simulink model "SMPC_safeconstr"  (R2024b)
settings: Solver=ode4  StartTime=0.0  StopTime=tsim  FixedStep=baseRate  RelTol=1e-6  AbsTol=1e-6
values from neighbouring files (symbols this model uses):
  C = [cos(theta), -sin(theta) ... (first row only)    [Run_Initializer.m]
  docking_face = [0 1]'    [Run_Initializer.m]
  docking_offset = [0 0 0]'    [Run_Initializer.m]
  eta = 0.7    [Run_Initializer.m]
  F_t = [kron(eye(N_h),  [zeros(2,3), eye(2), zeros(2,4)]) ... (first row only)    [Run_Initializer.m]
  f_t = [kron(ones(N_h, 1), [xLength yLength]' - edge_buffer) ... (first row only)    [Run_Initializer.m]
  F_u = [kron(eye(N_h),  [eye(3), zeros(3,6)]) ... (first row only)    [Run_Initializer.m]
  f_u = kron(ones(2*N_h, 1), u_max')    [Run_Initializer.m]
  gamma = 0.95    [Run_Initializer.m]
  Gamma1_el = 0.12    [Run_Initializer.m]
  Gamma1_sh = 0.005    [Run_Initializer.m]
  Gamma1_wr = 0.025    [Run_Initializer.m]
  Gamma2_el = 5    [Run_Initializer.m]
  Gamma2_sh = 5    [Run_Initializer.m]
  Gamma2_wr = 5    [Run_Initializer.m]
  Gamma3_el = 10    [Run_Initializer.m]
  Gamma3_sh = 40    [Run_Initializer.m]
  Gamma3_wr = 40    [Run_Initializer.m]
  Gamma4_el = 0.039    [Run_Initializer.m]
  Gamma4_sh = 0.015    [Run_Initializer.m]
  Gamma4_wr = 0.029    [Run_Initializer.m]
  Gamma5_el = 800    [Run_Initializer.m]
  Gamma5_sh = 800    [Run_Initializer.m]
  Gamma5_wr = 800    [Run_Initializer.m]
  Gamma6_el = 0.000001    (= 1e-06)    [Run_Initializer.m]
  Gamma6_sh = 0.005    [Run_Initializer.m]
  Gamma6_wr = 0.02    [Run_Initializer.m]
  H = kron(eye(N_h), [R, zeros(3,6); zeros(6,3), Q])    [Run_Initializer.m]
  Kd_elarm = 0.8    [Run_Initializer.m]
  Kd_sharm = 1.0    (= 1)    [Run_Initializer.m]
  Kd_wrarm = 0.6    [Run_Initializer.m]
  Kp_elarm = 1.2    [Run_Initializer.m]
  Kp_sharm = 1.5    [Run_Initializer.m]
  Kp_wrarm = 1.0    (= 1)    [Run_Initializer.m]
  lambda = (alpha^2)*(6 + kappa) - 6    (= 15.06)    [Run_Initializer.m]
  PWMFreq = 5    [Run_Initializer.m]
  Q_k = [1e-6*eye(3)  zeros(3,3) ... (first row only)    [Run_Initializer.m]
  r_hold_min = [0.8; (0.3+0.05)]    [Run_Initializer.m]
  r_hold_obs = 1.1*sqrt(2)*0.3.*[1;1]    [Run_Initializer.m]
  R_k = diag([0.02^2 0.02^2 0.01^2])    [Run_Initializer.m]
  T_d = 2    [Run_Initializer.m]
  Tz_lim_elarm = .1    (= 0.1)    [Run_Initializer.m]
  Tz_lim_sharm = .1    (= 0.1)    [Run_Initializer.m]
  Tz_lim_wrarm = .1    (= 0.1)    [Run_Initializer.m]
  use_table_constr = false    [Run_Initializer.m]
  w_c = [w_c0, w_i.*ones(1, 2*6)]    [Run_Initializer.m]
  w_m = [w_m0, w_i.*ones(1, 2*6)]    [Run_Initializer.m]
  x_BLACK_0 = [0.32 0.32 315*d2r 0.01 0.005 1*d2r]'    [Run_Initializer.m]
  x_BLUE_0 = [0.5 0.5 315*d2r 0.01 0.01 1*d2r]'    [Run_Initializer.m]
  x_obs_0 = [x_BLUE_0(1:3) + diag(sqrt(R_k)); 0.01; 0.01; 0.005]    [Run_Initializer.m]
  x_tar_0 = [x_BLACK_0(1:3) + diag(sqrt(R_k)); 0.01; 0.01; 0.005]    [Run_Initializer.m]
  zeta = 10*d2r    (= 0.174532925199)    [Run_Initializer.m]
undefined symbols (not defined in the file or in its folder): a1, a2, a3, b0, b1, b2, b3, baseRate, camera_FOV, camera_offset, dataRate, DiscIntNeverNeededParam, drop_states_ARM, drop_states_BLACK, drop_states_BLUE, drop_states_RED, F_black_X_nominal, F_black_Y_nominal, F_blue_X_nominal, F_blue_Y_nominal, F_red_X_nominal, F_red_Y_nominal, F_thrusters_BLACK, F_thrusters_BLUE, F_thrusters_RED, home_states_BLACK, home_states_BLUE, home_states_RED, IBLACK, IBLUE, IDIST, IEE, init_states_BLACK, init_states_BLUE, init_states_RED, IPROX, IRED, K_BLACK, K_BLUE, K_RED, Kd_tb, Kd_tblue, Kd_tr, Kd_xb, Kd_xblue, Kd_xr, Kd_yb, Kd_yblue, Kd_yr, Kp_tb, Kp_tblue, Kp_tr, Kp_xb, Kp_xblue, Kp_xr, Kp_yb, Kp_yblue, Kp_yr, mBLACK, mBLUE ... (+23)
libraries: simulink x30, nvidiaSharedBlocks x12, dspsigops x7, MainLibrary x5, dspinverses x3, nvidiaIMUSensorslib x1
(part 7 of 8)

== matlab function SMPC_safeconstr/PhaseSpace Camera Code/Use Hardware to Obtain States/Store BLACK Data/Subsystem2/Enabled Subsystem/MATLAB Function ==
  data: y input; dy output; dt input; tau input; dy_prev input; ema_prev input; ema output
function [dy, ema] = realtime_derivative_ema(y, dt, tau, dy_prev, ema_prev)
    % Inputs:
    % y: Current measurement
    % dt: Time step
    % alpha: Smoothing factor (e.g., 0.1)

    alpha = 1 - exp(-dt / tau);
        
    % Update EMA
    ema = alpha.*y + (1 - alpha).*ema_prev;
    
    % Compute derivative
    dy = (ema - ema_prev)./dt;
    
end

== matlab function SMPC_safeconstr/PhaseSpace Camera Code/Use Hardware to Obtain States/Store BLUE Data/Calculate True Time Step/MATLAB Function ==
  data: dt input; dt_out output; dataRate input
function dt_out = CheckforInvalidTime(dt, dataRate)

    if dt <= 0

        dt_out = dataRate;

    else

        dt_out = dt;

    end


end

== matlab function SMPC_safeconstr/PhaseSpace Camera Code/Use Hardware to Obtain States/Store BLUE Data/Subsystem1/Enabled Subsystem/MATLAB Function ==
  data: y input; dy output; dt input; tau input; dy_prev input; ema_prev input; ema output
function [dy, ema] = realtime_derivative_ema(y, dt, tau, dy_prev, ema_prev)
    % Inputs:
    % y: Current measurement
    % dt: Time step
    % alpha: Smoothing factor (e.g., 0.1)

    alpha = 1 - exp(-dt / tau);
        
    % Update EMA
    ema = alpha.*y + (1 - alpha).*ema_prev;
    
    % Compute derivative
    dy = (ema - ema_prev)./dt;
    
end

== matlab function SMPC_safeconstr/PhaseSpace Camera Code/Use Hardware to Obtain States/Store BLUE Data/Subsystem2/Enabled Subsystem/MATLAB Function ==
  data: y input; dy output; dt input; tau input; dy_prev input; ema_prev input; ema output
function [dy, ema] = realtime_derivative_ema(y, dt, tau, dy_prev, ema_prev)
    % Inputs:
    % y: Current measurement
    % dt: Time step
    % alpha: Smoothing factor (e.g., 0.1)

    alpha = 1 - exp(-dt / tau);
        
    % Update EMA
    ema = alpha.*y + (1 - alpha).*ema_prev;
    
    % Compute derivative
    dy = (ema - ema_prev)./dt;
    
end

== matlab function SMPC_safeconstr/Simulate Plant Dynamics/RED and ARM Dynamics/RED Only/Dynamics Model for RED/MATLAB Function ==
  data: control_inputs input; x_ddot output; mRED parameter; IRED parameter

    function x_ddot = RED_dynamics(control_inputs, mRED, IRED)

        %#codegen
        % Fully define the size of x_ddot() for code generation:
        x_ddot     = zeros(3,1);

        % Extract the servicer model parameters from the model_param vector defined
        % in initialize.m:

        % Extract the control inputs from the control_input vector:
        Fx        = control_inputs(1);              % [N]
        Fy        = control_inputs(2);              % [N]
        Tz        = control_inputs(3);              % [N.m]

        % Calculate the state acceleration vector:
        x_ddot(1) = Fx/mRED;                      % [m/s^2]
        x_ddot(2) = Fy/mRED;                      % [m/s^2]
        x_ddot(3) = Tz/IRED;                      % [rad/s^2]

    end

== matlab function SMPC_safeconstr/Stochastic Model Predictive Control/Stochastic Model Predictive Control/Execute quadprog ==
  data: z_t input; P input; h input; H parameter; b input; z output; z_0 input; u output; C parameter; result output
% Solve the linear-quadratic optimization problem
function [z, u, result] = fcn(z_t, P, h, H, b, z_0, C)

% Compute equivalent cost function matrices
f = (-2.*z_t'*H)';
H = 2.*H;

% Configure solver options
options = optimoptions('quadprog', 'Algorithm', 'active-set', 'MaxIterations', 300);

% Call solver and time it
tic
[z, ~, exitflag, output] = quadprog(H, f, P, h, C, b, [], [], z_0, options);
cputime = toc;

% Output solver results
result = [exitflag, output.iterations, cputime];

% Extract optimized control input for the current step
u = z(1:3);

== matlab function SMPC_safeconstr/Stochastic Model Predictive Control/Stochastic Model Predictive Control/Propogate BLACK trajectory ==
  data: x_BLACK input; z_BLACK output; T_d parameter
% Compute expected trajectory of the target spacecraft
function z_BLACK = fcn(x_BLACK, T_d)

% Define horizon length
N_h = 15;

% Pre-allocate target trajectory variable
z_BLACK = zeros(9*N_h,1);

% Extract target velocities (assume constant velocity over the horizon)
v_BLACK = x_BLACK(4:6);

% Compute first entry with initial position
z_BLACK(4:9) = [x_BLACK(1:3) + v_BLACK.*T_d; v_BLACK];

% Iterate over the horizon
for j = 2:N_h
    row = 9*(j-1)+1;

    % Extract prior position
    pos_BLACK = z_BLACK(row-9+3:row-9+5);

    % Insert propogated position
    z_BLACK(row+3:row+9-1) = [pos_BLACK + v_BLACK.*T_d; v_BLACK];
end

end

== matlab function SMPC_safeconstr/Stochastic Model Predictive Control/Stochastic Model Predictive Control/Propogate BLUE trajectory ==
  data: x_BLUE input; z_BLUE output; T_d parameter
% Compute expected trajectory of the target spacecraft
function z_BLUE = fcn(x_BLUE, T_d)

% Define horizon length
N_h = 15;

% Pre-allocate target trajectory variable
z_BLUE = zeros(9*N_h,1);

% Extract target velocities (assume constant velocity over the horizon)
v_BLUE = x_BLUE(4:6);

% Compute first entry with initial position
z_BLUE(4:9) = [x_BLUE(1:3) + v_BLUE.*T_d; v_BLUE];

% Iterate over the horizon
for j = 2:N_h
    row = 9*(j-1)+1;

    % Extract prior position
    pos_BLUE = z_BLUE(row-9+3:row-9+5);

    % Insert propogated position
    z_BLUE(row+3:row+9-1) = [pos_BLUE + v_BLUE.*T_d; v_BLUE];
end

end

== matlab function SMPC_safeconstr/Simulate Plant Dynamics/RED and ARM Dynamics/RED + ARM/Data @ Measurement Rate/Calculate True Time Step/MATLAB Function ==
  data: dt input; dt_out output; dataRate input
function dt_out = CheckforInvalidTime(dt, dataRate)

    if dt <= 0

        dt_out = dataRate;

    else

        dt_out = dt;

    end


end

== matlab function SMPC_safeconstr/Simulate Plant Dynamics/RED and ARM Dynamics/RED + ARM/Calculated & Store Measured States/Subsystem3/Enabled Subsystem/MATLAB Function ==
  data: y input; dy output; dt input; tau input; dy_prev input; ema_prev input; ema output
function [dy, ema] = realtime_derivative_ema(y, dt, tau, dy_prev, ema_prev)
    % Inputs:
    % y: Current measurement
    % dt: Time step
    % alpha: Smoothing factor (e.g., 0.1)

    alpha = 1 - exp(-dt / tau);
        
    % Update EMA
    ema = alpha.*y + (1 - alpha).*ema_prev;
    
    % Compute derivative
    dy = (ema - ema_prev)./dt;
    
end

== matlab function SMPC_safeconstr/Stochastic Model Predictive Control/Stochastic Model Predictive Control/Update Holding Radius ==
  data: r_hold input; x_RED input; x_BLACK input; r_hold_min parameter; eta parameter; zeta parameter; gamma parameter; docking_face parameter; r_hold output; docking_offset parameter; docking input; docking output
% Compute next holding radius
function [r_hold, docking] = fcn(r_hold, x_RED, x_BLACK, r_hold_min, eta, zeta, gamma, docking_face, docking_offset, docking)

% Compute 2D z-axis rotation matrix representing the targets attitude
R = [cos(x_BLACK(3)) -sin(x_BLACK(3)); sin(x_BLACK(3)) cos(x_BLACK(3))];

% Compute the docking position in the global frame relative to the target
r_dock = R*(r_hold(2).*docking_face + docking_offset(1:2));

% Compute the required attitude for docking
theta_star = x_BLACK(3) + docking_offset(3)-pi/2;

% Compute required chaser state for docking
x_t = [x_BLACK(1:2) + r_dock; theta_star];

% Compute positional and attitude errors
x_error = (x_RED(1:2) - x_t(1:2))'*(x_RED(1:2) - x_t(1:2));
theta_error = abs(atan2(sin(x_RED(3) - x_t(3)), cos(x_RED(3) - x_t(3))));

% Scale holding radius if tolerances are met
if x_error < eta^2 && theta_error < zeta
    r_hold = gamma*r_hold;
    docking = 1;
end

% Ensure holding radius does go below the defined minimum radius
r_hold = max(r_hold, r_hold_min);

end

== matlab function SMPC_safeconstr/Simulate Plant Dynamics/RED and ARM Dynamics/RED + ARM/Calculated & Store Measured States/Subsystem4/Enabled Subsystem/MATLAB Function ==
  data: y input; dy output; dt input; tau input; dy_prev input; ema_prev input; ema output
function [dy, ema] = realtime_derivative_ema(y, dt, tau, dy_prev, ema_prev)
    % Inputs:
    % y: Current measurement
    % dt: Time step
    % alpha: Smoothing factor (e.g., 0.1)

    alpha = 1 - exp(-dt / tau);
        
    % Update EMA
    ema = alpha.*y + (1 - alpha).*ema_prev;
    
    % Compute derivative
    dy = (ema - ema_prev)./dt;
    
end

== matlab function SMPC_safeconstr/Simulate Plant Dynamics/RED and ARM Dynamics/RED + ARM/Calculated & Store Measured States/Subsystem5/Enabled Subsystem/MATLAB Function ==
  data: y input; dy output; dt input; tau input; dy_prev input; ema_prev input; ema output
function [dy, ema] = realtime_derivative_ema(y, dt, tau, dy_prev, ema_prev)
    % Inputs:
    % y: Current measurement
    % dt: Time step
    % alpha: Smoothing factor (e.g., 0.1)

    alpha = 1 - exp(-dt / tau);
        
    % Update EMA
    ema = alpha.*y + (1 - alpha).*ema_prev;
    
    % Compute derivative
    dy = (ema - ema_prev)./dt;
    
end

== matlab function SMPC_safeconstr/Stochastic Model Predictive Control/Unscented Kalman Filter (TARGET)/Unscented Kalman Filter ==
  data: x_0 input; P_0 input; z input; x_est output; P_est output; baseRate parameter; Q_k parameter; R_k parameter; lambda parameter; w_m parameter; w_c parameter
function [x_est, P_est] = fcn(x_0, P_0, z, baseRate, Q_k, R_k, lambda, w_m, w_c)
    % Define dynamics model (using forward euler integration)
    dynamics = @(x, dt) x + dt.*[x(4:6); zeros(3,1)];

    % Define measurement model
    measure = @(x) x(1:3);

    % Run a step of the UKF
    [x_est, P_est] = estimate_UKF(x_0, P_0, z, baseRate, dynamics, measure, ...
                                  6, Q_k, R_k, lambda, w_m, w_c, 3);
end

%% Unscented Kalman Filter Estimation
function [x_est, P_est] = estimate_UKF(x_0, P_0, z, dt, dynamics_fcn, measure_fcn, N, Q, R, lambda, w_m, w_c, d_max)
    % Compute the cholesky decomposition
    L = chol((N + lambda)*P_0)';
    
    % Place sigma points
    X = [x_0, x_0 + L, x_0 - L];
    
    % Propogate sigma points through the dynamics model
    X_plus = zeros(size(X));
    for i = 1:size(X,2)
        X_plus(:,i) = dynamics_fcn(X(:,i), dt);
    end

    % Compute the predicted state and covariance
    x_bar = X_plus*w_m';
    P_bar = (X_plus - x_bar)*diag(w_c)*(X_plus - x_bar)' + Q;

    % Transfer sigma points into the measurement space
    Z = zeros(size(z,1), size(X,2));
    for i = 1:size(X,2)
        Z(:,i) = measure_fcn(X_plus(:,i));
    end

    % Compute the predicted measurement
    z_bar = Z*w_m';

    % Compute measurement covariance and state-measurement cross-covariance
    P_zz = (Z - z_bar)*diag(w_c)*(Z - z_bar)' + R;
    P_xz = (X_plus - x_bar)*diag(w_c)*(Z - z_bar)';

    % Compute the residue
    y = z - z_bar;

    if anynan(z) || all(z == 0) || y'*P_zz*y >= d_max^2
        % If there is no measurement, or it is an outlier, use prediction only
        x_est = x_bar;
        P_est = P_bar;
    else
        % Compute the kalman gain
        % K = P_xz/P_zz;
        K = P_xz*inv(P_zz);

        % Compute estimated state and covariance
        x_est = x_bar + K*y;
        P_est = P_bar - K*P_zz*K';
    end
end

== matlab function SMPC_safeconstr/Stochastic Model Predictive Control/Stochastic Model Predictive Control/Obstacle Collision Constraint ==
  data: r_hold_obs parameter; z_BLUE input; F_c output; z_RED input; f_c output; platformSelection parameter; P input
function [F_c, f_c] = fcn(r_hold_obs, z_BLUE, z_RED, platformSelection, P)

% Define horizon length
N_h = 15;

% Define shape matrix
S = diag(r_hold_obs.^-2);

% Pre-allocate expansion point position vector over the horizon
r_0_bar = zeros(9*N_h,1);

% Pre-allocate D matrix
F_c = zeros(N_h, 9*N_h);
f_c = zeros(N_h,1);

alpha = zeros(N_h,1);

if platformSelection >= 6 && platformSelection <= 11
    
    % Iterate over the horizon
    for j = 1:N_h
        pos = 9*(j-1)+1;
        
        % Extract target & chaser positions, and target attitude
        r_obs = z_BLUE(pos+3:pos+4);
        r_chs = z_RED(pos+3:pos+4);
        theta_tar = z_BLUE(pos+5);
    
        % Compute target -> chaser unit vector
        u_tc = (r_chs-r_obs)/norm(r_chs-r_obs);
    
        % Compute target body-fixed -> inertial rotation matrix
        R = [cos(theta_tar) -sin(theta_tar); 
             sin(theta_tar) cos(theta_tar)];
    
        % Compute angle between target-chaser vector and target body-fixed
        % x-axis in inertial frame
        theta_e = acos(u_tc'*(R*[1; 0]));
    
        % Extract semi-(major/minor) axes
        [a_e, b_e] = deal(r_hold_obs(1), r_hold_obs(2));
    
        % Compute ellipse radius at current angle
        r_e = a_e*b_e/sqrt((a_e*sin(theta_e))^2 + (b_e*cos(theta_e))^2);
    
        % Compute expansion point position
        r_0 = r_obs + r_e.*u_tc;
    
        % Store expansion point positions in respective vector
        r_0_bar(pos+3:pos+4) = r_0;
    
        % Configure solver options
        options = optimoptions('quadprog', 'Algorithm', 'active-set', 'MaxIterations', 300);

        w = diag(P(1:2,1:2));

        % Call solver and time it
        w_opt = quadprog(2.*(R*S*R'), (2.*(r_obs-r_chs)'*(R*S*R'))', [], [], [], [], -w, w, [0 0], options);
        alpha(j) = w_opt'*(R*S*R')*w_opt+2*(r_obs-r_chs)'*(R*S*R')*w_opt;

        % Compute E matrix
        E = (r_0-r_obs)'*(R*S*R');
    
        row = j;
        col = 3+9*(j-1)+1;
        
        F_c(row,col:col+1) = -2.*E;
        f_c(row,1) = -1-E*(r_0+r_obs); %+ alpha(j);
    
    end
end

end

== matlab function SMPC_safeconstr/2 - Guidance/Default APF PPL (BLACK)/MATLAB Function ==
  data: desiredPosition input; currentPosition output; currentPosition input; obstacles input; attractiveGain input; repulsiveGain input; influenceRange input; angularGain input; baseRate parameter
function currentPosition = APFPathPlanner(desiredPosition, currentPosition, obstacles, attractiveGain, repulsiveGain, influenceRange, angularGain, baseRate)
    % APFPathPlanner for real-time path planning in Simulink
    % Controls X, Y, and Attitude (Theta)
    % currentPosition: [x, y, theta]
    % desiredPosition: [x, y, theta]
    % obstacles: Nx2 matrix of obstacle positions [x, y]
    % attractiveGain: Scalar for attractive force
    % repulsiveGain: Scalar for repulsive force
    % influenceRange: Scalar, range for obstacle influence
    % angularGain: Scalar for angular adjustment


    % Position control for X and Y
    attractiveForce = attractiveGain * (desiredPosition(1:2) - currentPosition(1:2));
    repulsiveForce = zeros(1, 2);

    % % Repulsive force from obstacles
    for i = 1:size(obstacles, 1)
        obstaclePos = obstacles(i, :);
        distanceToObstacle = norm(currentPosition(1:2) - obstaclePos);

        if distanceToObstacle < influenceRange
            directionFromObstacle = (currentPosition(1:2) - obstaclePos) / distanceToObstacle;
            magnitude = repulsiveGain * (1 / distanceToObstacle - 1 / influenceRange) * (1 / distanceToObstacle^2);
            repulsiveForce = repulsiveForce + magnitude * directionFromObstacle;
        end
    end

    % Combine attractive and repulsive forces
    totalForce = attractiveForce + repulsiveForce;

    % Update X and Y position
    deltaT = baseRate;
    newPosition = currentPosition(1:2) + deltaT * totalForce;

    % Attitude control for Theta
    angularDifference = atan2(sin(desiredPosition(3) - currentPosition(3)), cos(desiredPosition(3) - currentPosition(3)));
    newTheta = currentPosition(3) + angularGain * angularDifference * deltaT;

    % Normalize newTheta to be within -pi to pi
    newTheta = atan2(sin(newTheta), cos(newTheta));

    % Update currentPosition with new position and attitude
    currentPosition = [newPosition, newTheta];

end

== matlab function SMPC_safeconstr/Stochastic Model Predictive Control/Stochastic Model Predictive Control/Target Vision Constraint ==
  data: z_BLACK input; z_RED input; docking input; f_v output; docking_offset parameter; camera_FOV parameter; camera_offset parameter
 function f_v = fcn(z_BLACK, z_RED, docking, docking_offset, camera_FOV, camera_offset)

% Define horizon length
N_h = 15;

% Pre-allocate p vector
f_v = zeros(2*N_h,1);

% Iterate over the horizon
for j = 1:N_h
    pos = 9*(j-1)+1;

    R = [cos(z_RED(pos+5)), -sin(z_RED(pos+5)); 
         sin(z_RED(pos+5)),  cos(z_RED(pos+5))];

    % Compute relative position vector from camera to target
    r = z_BLACK(pos+3:pos+4) - z_RED(pos+3:pos+4) + R*camera_offset;

    % Compute desired pointing angle
    theta_star = rotateToFace(z_RED(pos+5), r) + docking_offset(3);

    if docking
        f_v(j) = theta_star + pi;
        f_v(j+N_h) = -1*(theta_star - pi);
    else
        f_v(j) = theta_star + (camera_FOV/2);
        f_v(j+N_h) = -1*(theta_star - (camera_FOV/2));
    end
end

end

%% Functions

function theta_des = rotateToFace(theta, r)
    theta_des = theta + wrapToPi(atan2(r(2),r(1)) - theta);
end

== matlab function SMPC_safeconstr/Thruster Control Code/Change BLACK Behavior/Calculate Duty Cycle/Generate Initial Guess/MATLAB Function ==
  data: H output; thruster_dist2CG_BLACK parameter; F_thrusters_BLACK parameter
function H = MakeH(thruster_dist2CG_BLACK,F_thrusters_BLACK)

    Vec1 = [ -1
             -1
              0 
              0
              1
              1
              0
              0 ];
          
    Vec2 = [  0
              0
              1
              1
              0
              0
             -1
             -1 ];
         
    Vec3 = thruster_dist2CG_BLACK./1000;
    
    Mat1 = [Vec1, Vec2, Vec3]';
    
    Mat2 = diag((F_thrusters_BLACK./2));
    
    H    = Mat1*Mat2;

end

== matlab function SMPC_safeconstr/Corrupt Ground Truth/Custom Noise Generator ==
  data: y output; u parameter; v parameter
function y = fcn(u, v)
    if length(u) ~= length(v)
        error('The length of the means and variances must be the same')
    end
    
    y = u + sqrt(v).*randn(length(u),1);
end

== matlab function SMPC_safeconstr/Thruster Control Code/Change BLACK Behavior/Calculate Duty Cycle/MATLAB Function1 ==
  data: ThrustPer_Final output; ThrustPer input; PWMFreq parameter
function ThrustPer_Final  = ThrusterSat(ThrustPer, PWMFreq)

    ValveTime       = 0.007;
    TControl        = 1/PWMFreq;

    ThrustPer_Final = zeros(8,1);
    
    if max(ThrustPer) > 1
        ThrustPer_Sat = ThrustPer/max(ThrustPer);
    else
        ThrustPer_Sat = ThrustPer;
    end
    
    for i = 1:8
        if ThrustPer_Sat(i) > ValveTime/TControl 
            ThrustPer_Final(i) = ThrustPer_Sat(i);
        else
            %ThrustPer_Final(i) = 0;
        end
    end


end

== matlab function SMPC_safeconstr/Corrupt Ground Truth/Custom Noise Generator1 ==
  data: y output; u parameter; v parameter
function y = fcn(u, v)
    if length(u) ~= length(v)
        error('The length of the means and variances must be the same')
    end
    
    y = u + sqrt(v).*randn(length(u),1);
end

== matlab function SMPC_safeconstr/Stochastic Model Predictive Control/Stochastic Model Predictive Control/Compute Target Trajectory ==
  data: r_hold input; z_RED input; z_BLACK input; docking input; docking_face parameter; z_t output; docking_offset parameter
% Compute docking position over the horizon
function z_t  = fcn(r_hold, z_RED, z_BLACK, docking, docking_face, docking_offset)

% Define horizon length
N_h = 15;

% Pre-allocate target trajectory vector
z_t = zeros(9*N_h,1);

% Iterate over the horizon
for j = 1:N_h
    pos = 9*(j-1)+1;
    % Compute 2D z-axis rotation matrix representing the targets attitude
    R = rotz(z_BLACK(pos+5));

    % Compute the docking position in the global frame relative to the target
    r_dock = R*(r_hold(2).*docking_face + docking_offset(1:2));

    % Compute the required attitude for docking
        
    theta_star = z_BLACK(pos+5) + docking_offset(3)-pi/2;
    
    % Store required attitude and position for docking
    z_t(pos+3:pos+4) = z_BLACK(pos+3:pos+4) + r_dock;
    z_t(pos+5) = theta_star;
end

end

%% Functions

function C = rotz(theta)
    C = [cos(theta) -sin(theta); sin(theta) cos(theta)];
end

function theta_des = rotateToFace(theta, r)
    theta_des = theta + wrapToPi(atan2(r(2),r(1)) - theta);
end

== matlab function SMPC_safeconstr/Stochastic Model Predictive Control/Stochastic Model Predictive Control/Dynamic Target Collision Constraint ==
  data: r_hold input; z_BLACK input; F_h output; z_RED input; f_h output; P input
function [F_h, f_h] = fcn(r_hold, z_BLACK, z_RED, P)

% Define horizon length
N_h = 15;

% Define shape matrix
S = diag(r_hold.^-2);

% Pre-allocate expansion point position vector over the horizon
r_0_bar = zeros(9*N_h,1);

% Pre-allocate D matrix
F_h = zeros(N_h, 9*N_h);
f_h = zeros(N_h,1);

alpha = zeros(N_h,1);

% Iterate over the horizon
for j = 1:N_h
    pos = 9*(j-1)+1;
    
    % Extract target & chaser positions, and target attitude
    r_tar = z_BLACK(pos+3:pos+4);
    r_chs = z_RED(pos+3:pos+4);
    theta_tar = z_BLACK(pos+5);

    % Compute target -> chaser unit vector
    u_tc = (r_chs-r_tar)/norm(r_chs-r_tar);

    % Compute target body-fixed -> inertial rotation matrix
    R = [cos(theta_tar) -sin(theta_tar); 
         sin(theta_tar) cos(theta_tar)];

    % Compute angle between target-chaser vector and target body-fixed
    % x-axis in inertial frame
    theta_e = acos(u_tc'*(R*[1; 0]));

    % Extract semi-(major/minor) axes
    [a_e, b_e] = deal(r_hold(1), r_hold(2));

    % Compute ellipse radius at current angle
    r_e = a_e*b_e/sqrt((a_e*sin(theta_e))^2 + (b_e*cos(theta_e))^2);

    % Compute expansion point position
    r_0 = r_tar + r_e.*u_tc;

    % Store expansion point positions in respective vector
    r_0_bar(pos+3:pos+4) = r_0;

    % Configure solver options
    options = optimoptions('quadprog', 'Algorithm', 'active-set', 'MaxIterations', 300);
    
    w = diag(P(1:2,1:2));

    % Call solver and time it
    w_opt = quadprog(2.*(R*S*R'), (2.*(r_tar-r_chs)'*(R*S*R'))', [], [], [], [], -w, w, [0 0], options);
    alpha(j) = w_opt'*(R*S*R')*w_opt+2*(r_tar-r_chs)'*(R*S*R')*w_opt;

    % Compute E matrix
    E = (r_0-r_tar)'*(R*S*R');

    row = j;
    col = 3+9*(j-1)+1;

    F_h(row,col:col+1) = -2.*E;
    f_h(row) = -1-E*(r_0+r_tar);% + alpha(j);

end

r_tar = z_BLACK(4:5);
r_chs = z_RED(4:5);
u_tc = (r_chs-r_tar)/norm(r_chs-r_tar);

out = [f_h(1) r_tar' u_tc' z_BLACK(6) alpha(1)];

end

== matlab function SMPC_safeconstr/Stochastic Model Predictive Control/Stochastic Model Predictive Control/Shift Optimization Variable ==
  data: z input; z_0 output
function z_0 = fcn(z)

% Shift reference trajectory by dropping first control input and state,
% set last control input as zeros and duplicate last state
z_0 = [z(9+1:end); zeros(3,1); z(end-5:end)];

end

== matlab function SMPC_safeconstr/Thruster Control Code/Change BLACK Behavior/Calculate Duty Cycle/MATLAB Function5 ==
  data: H_final output; u_desired input; duty_cycles output; x0 input; thruster_dist2CG_BLACK parameter; F_black_X_nominal parameter; F_black_Y_nominal parameter; max_iters parameter; tol parameter
function [H_final,duty_cycles] = optimize_duty_cycle_with_decay(u_desired, x0, thruster_dist2CG_BLACK, F_black_X_nominal, F_black_Y_nominal, max_iters, tol)
    % Optimizes thruster duty cycles with decay factor updates
    %
    % Inputs:
    %   u_desired - Desired force and torque vector [Fx; Fy; M] (3x1)
    %   x0 - Initial guess for duty cycles (vector, 8x1)
    %   max_iters - Maximum number of iterations for convergence
    %   tol - Convergence tolerance for duty cycles
    %   thruster_dist2CG_BLACK - Distances of thrusters from CG (vector, mm)
    %   F_red_X_nominal - Nominal X thruster force (scalar, N)
    %   F_red_Y_nominal - Nominal Y thruster force (scalar, N)
    %
    % Outputs:
    %   duty_cycles - Optimal duty cycles for each thruster (vector, 8x1)

    % Initialization
    num_thrusters = length(x0);
    duty_cycles = x0; % Start with the initial guess
    thrust_decay_factor = 1; % Initial decay factor
    prev_duty_cycles = duty_cycles + 2 * tol; % Ensure loop starts

    % Iterative optimization process
    for iter = 1:max_iters
        % Update H matrix based on the current decay factor
        H = MakeHWithDecay(thruster_dist2CG_BLACK, F_black_X_nominal, thrust_decay_factor, F_black_Y_nominal);
        
        % Define quadratic programming problem
        Q = 2 * (H' * H); % Quadratic term
        c = -2 * (H' * u_desired); % Linear term
        lb = zeros(num_thrusters, 1); % Lower bounds
        ub = ones(num_thrusters, 1); % Upper bounds
        options = optimoptions('quadprog', 'Display', 'off', 'Algorithm', 'active-set', 'MaxIterations', 5);
        
        % Solve for optimal duty cycles
        [duty_cycles, ~, ~] = quadprog(Q, c, [], [], [], [], lb, ub, duty_cycles, options);
        
        % Update decay factor based on the current duty cycles
        [thrust_decay_factor, ~] = check_thrust_decay(duty_cycles);
                
        % Check convergence criteria
        if norm(duty_cycles - prev_duty_cycles, Inf) < tol
            H_final = MakeHWithDecayRecalculateForce(thruster_dist2CG_BLACK, F_black_X_nominal, thrust_decay_factor, F_black_Y_nominal);
            return;
        end
            
        
        % Update for next iteration
        prev_duty_cycles = duty_cycles;
    end
    
    H_final = MakeHWithDecayRecalculateForce(thruster_dist2CG_BLACK, F_black_X_nominal, thrust_decay_factor, F_black_Y_nominal);
   

end

function H = MakeHWithDecay(thruster_dist2CG, F_X_nominal, thrust_decay_factor, F_Y_nominal)
    % Constructs the H matrix with thrust decay adjustments
    %
    % Inputs:
    %   thruster_dist2CG - Distances of thrusters from CG (vector, mm)
    %   F_X_nominal - Nominal X thruster force (scalar, N)
    %   thrust_decay_factor - Decay factor for thrust (scalar)
    %   F_Y_nominal - Nominal Y thruster force (scalar, N)
    %
    % Output:
    %   H - H matrix for optimization (3x8)

    % Adjust thruster distances (convert to meters)
    adjusted_thruster_dist2CG = thruster_dist2CG / 1000;

    % Define thruster contribution vectors
    Vec1 = [-1; -1;  0;  0;  1;  1;  0;  0]; % X-component
    Vec2 = [ 0;  0;  1;  1;  0;  0; -1; -1]; % Y-component
    Vec3 = adjusted_thruster_dist2CG;        % Moment arm (Z)

    % Combine vectors into the H matrix structure
    Mat1 = [Vec1, Vec2, Vec3]';
    
    % Adjust thruster forces with decay factor
    F_thrusters = [F_X_nominal; F_X_nominal; F_Y_nominal; F_Y_nominal; 
                   F_X_nominal; F_X_nominal; F_Y_nominal; F_Y_nominal] * thrust_decay_factor;

    % Scale forces for H matrix
    Mat2 = diag(F_thrusters / 2);

    % Compute final H matrix
    H = Mat1 * Mat2;
end

function H = MakeHWithDecayRecalculateForce(thruster_dist2CG, F_X_nominal, thrust_decay_factor, F_Y_nominal)
    % Constructs the H matrix with thrust decay adjustments
    %
    % Inputs:
    %   thruster_dist2CG - Distances of thrusters from CG (vector, mm)
    %   F_X_nominal - Nominal X thruster force (scalar, N)
    %   thrust_decay_factor - Decay factor for thrust (scalar)
    %   F_Y_nominal - Nominal Y thruster force (scalar, N)
    %
    % Output:
    %   H - H matrix for optimization (3x8)

    % Adjust thruster distances (convert to meters)
    adjusted_thruster_dist2CG = thruster_dist2CG / 1000;

    % Define thruster contribution vectors
    Vec1 = [-1; -1;  0;  0;  1;  1;  0;  0]; % X-component
    Vec2 = [ 0;  0;  1;  1;  0;  0; -1; -1]; % Y-component
    Vec3 = adjusted_thruster_dist2CG;        % Moment arm (Z)

    % Combine vectors into the H matrix structure
    Mat1 = [Vec1, Vec2, Vec3]';
    
    % Adjust thruster forces with decay factor
    F_thrusters = [F_X_nominal; F_X_nominal; F_Y_nominal; F_Y_nominal; 
                   F_X_nominal; F_X_nominal; F_Y_nominal; F_Y_nominal] * thrust_decay_factor;

    % Scale forces for H matrix
    Mat2 = diag(F_thrusters);

    % Compute final H matrix
    H = Mat1 * Mat2;
end

function [thrust_decay_factor, count] = check_thrust_decay(PWMs)
    % Updates the thrust decay factor based on current duty cycles
    %
    % Inputs:
    %   PWMs - Current duty cycle values (vector)
    %
    % Outputs:
    %   thrust_decay_factor - Updated decay factor (scalar)
    %   count - Number of active thrusters (scalar)

    % Normalize PWMs if necessary
    if max(PWMs) > 1
        PWMs = PWMs / max(PWMs);
    end

    % Count active thrusters
    count = sum(PWMs > 0);
    
    % Compute average duty cycle for active thrusters
    average_duty_cycle_per_thruster = sum(max(PWMs, 0)) / max(count, 1);

    % Update thrust decay factor based on average duty cycle
    if average_duty_cycle_per_thruster < 0.3 || count == 0
        thrust_decay_factor = 1;
    else
        thrust_decay_factor = max(0.6 - 2 * average_duty_cycle_per_thruster + 1, 0.5);
    end
end

== matlab function SMPC_safeconstr/Thruster Control Code/Change BLACK Behavior/Calculate Duty Cycle/Rotate Forces to Inertial/Create Rotation Matrix ==
  data: Rz input; C_Ib output
function C_Ib = RotateFrame(Rz)

C_bI = [  cos(Rz) sin(Rz)
         -sin(Rz) cos(Rz) ];

C_Ib = inv(C_bI);

end

== matlab function SMPC_safeconstr/Thruster Control Code/Change BLACK Behavior/Rotate Forces to Body/Create Rotation Matrix ==
  data: Rz input; C_bI output
function C_bI = RotateFrame(Rz)

C_bI = [  cos(Rz) sin(Rz)
         -sin(Rz) cos(Rz) ];

end

== matlab function SMPC_safeconstr/Thruster Control Code/Change BLUE Behavior/Calculate Duty Cycle/Generate Initial Guess/MATLAB Function ==
  data: H output; thruster_dist2CG_BLUE parameter; F_thrusters_BLUE parameter
function H = MakeH(thruster_dist2CG_BLUE,F_thrusters_BLUE)

    Vec1 = [ -1
             -1
              0 
              0
              1
              1
              0
              0 ];
          
    Vec2 = [  0
              0
              1
              1
              0
              0
             -1
             -1 ];
         
    Vec3 = thruster_dist2CG_BLUE./1000;
    
    Mat1 = [Vec1, Vec2, Vec3]';
    
    Mat2 = diag((F_thrusters_BLUE./2));
    
    H    = Mat1*Mat2;

end

== matlab function SMPC_safeconstr/Thruster Control Code/Change BLUE Behavior/Calculate Duty Cycle/MATLAB Function1 ==
  data: ThrustPer_Final output; ThrustPer input; PWMFreq parameter
function ThrustPer_Final  = ThrusterSat(ThrustPer, PWMFreq)

    ValveTime       = 0.007;
    TControl        = 1/PWMFreq;

    ThrustPer_Final = zeros(8,1);
    
    if max(ThrustPer) > 1
        ThrustPer_Sat = ThrustPer/max(ThrustPer);
    else
        ThrustPer_Sat = ThrustPer;
    end
    
    for i = 1:8
        if ThrustPer_Sat(i) > ValveTime/TControl 
            ThrustPer_Final(i) = ThrustPer_Sat(i);
        else
            ThrustPer_Final(i) = 0;
        end
    end


end

== matlab function SMPC_safeconstr/Thruster Control Code/Change BLUE Behavior/Calculate Duty Cycle/MATLAB Function5 ==
  data: H_final output; u_desired input; duty_cycles output; x0 input; thruster_dist2CG_BLUE parameter; F_blue_X_nominal parameter; F_blue_Y_nominal parameter; max_iters parameter; tol parameter
function [H_final,duty_cycles] = optimize_duty_cycle_with_decay(u_desired, x0, thruster_dist2CG_BLUE, F_blue_X_nominal, F_blue_Y_nominal, max_iters, tol)
    % Optimizes thruster duty cycles with decay factor updates
    %
    % Inputs:
    %   u_desired - Desired force and torque vector [Fx; Fy; M] (3x1)
    %   x0 - Initial guess for duty cycles (vector, 8x1)
    %   max_iters - Maximum number of iterations for convergence
    %   tol - Convergence tolerance for duty cycles
    %   thruster_dist2CG_BLUE - Distances of thrusters from CG (vector, mm)
    %   F_red_X_nominal - Nominal X thruster force (scalar, N)
    %   F_red_Y_nominal - Nominal Y thruster force (scalar, N)
    %
    % Outputs:
    %   duty_cycles - Optimal duty cycles for each thruster (vector, 8x1)

    % Initialization
    num_thrusters = length(x0);
    duty_cycles = x0; % Start with the initial guess
    thrust_decay_factor = 1; % Initial decay factor
    prev_duty_cycles = duty_cycles + 2 * tol; % Ensure loop starts

    % Iterative optimization process
    for iter = 1:max_iters
        % Update H matrix based on the current decay factor
        H = MakeHWithDecay(thruster_dist2CG_BLUE, F_blue_X_nominal, thrust_decay_factor, F_blue_Y_nominal);
        
        % Define quadratic programming problem
        Q = 2 * (H' * H); % Quadratic term
        c = -2 * (H' * u_desired); % Linear term
        lb = zeros(num_thrusters, 1); % Lower bounds
        ub = ones(num_thrusters, 1); % Upper bounds
        options = optimoptions('quadprog', 'Display', 'off', 'Algorithm', 'active-set', 'MaxIterations', 5);
        
        % Solve for optimal duty cycles
        [duty_cycles, ~, ~] = quadprog(Q, c, [], [], [], [], lb, ub, duty_cycles, options);
        
        % Update decay factor based on the current duty cycles
        [thrust_decay_factor, ~] = check_thrust_decay(duty_cycles);
                
        % Check convergence criteria
        if norm(duty_cycles - prev_duty_cycles, Inf) < tol
            H_final = MakeHWithDecayRecalculateForce(thruster_dist2CG_BLUE, F_blue_X_nominal, thrust_decay_factor, F_blue_Y_nominal);
            return;
        end
            
        
        % Update for next iteration
        prev_duty_cycles = duty_cycles;
    end
    
    H_final = MakeHWithDecayRecalculateForce(thruster_dist2CG_BLUE, F_blue_X_nominal, thrust_decay_factor, F_blue_Y_nominal);
   

end

function H = MakeHWithDecay(thruster_dist2CG, F_X_nominal, thrust_decay_factor, F_Y_nominal)
    % Constructs the H matrix with thrust decay adjustments
    %
    % Inputs:
    %   thruster_dist2CG - Distances of thrusters from CG (vector, mm)
    %   F_X_nominal - Nominal X thruster force (scalar, N)
    %   thrust_decay_factor - Decay factor for thrust (scalar)
    %   F_Y_nominal - Nominal Y thruster force (scalar, N)
    %
    % Output:
    %   H - H matrix for optimization (3x8)

    % Adjust thruster distances (convert to meters)
    adjusted_thruster_dist2CG = thruster_dist2CG / 1000;

    % Define thruster contribution vectors
    Vec1 = [-1; -1;  0;  0;  1;  1;  0;  0]; % X-component
    Vec2 = [ 0;  0;  1;  1;  0;  0; -1; -1]; % Y-component
    Vec3 = adjusted_thruster_dist2CG;        % Moment arm (Z)

    % Combine vectors into the H matrix structure
    Mat1 = [Vec1, Vec2, Vec3]';
    
    % Adjust thruster forces with decay factor
    F_thrusters = [F_X_nominal; F_X_nominal; F_Y_nominal; F_Y_nominal; 
                   F_X_nominal; F_X_nominal; F_Y_nominal; F_Y_nominal] * thrust_decay_factor;

    % Scale forces for H matrix
    Mat2 = diag(F_thrusters / 2);

    % Compute final H matrix
    H = Mat1 * Mat2;
end

function H = MakeHWithDecayRecalculateForce(thruster_dist2CG, F_X_nominal, thrust_decay_factor, F_Y_nominal)
    % Constructs the H matrix with thrust decay adjustments
    %
    % Inputs:
    %   thruster_dist2CG - Distances of thrusters from CG (vector, mm)
    %   F_X_nominal - Nominal X thruster force (scalar, N)
    %   thrust_decay_factor - Decay factor for thrust (scalar)
    %   F_Y_nominal - Nominal Y thruster force (scalar, N)
    %
    % Output:
    %   H - H matrix for optimization (3x8)

    % Adjust thruster distances (convert to meters)
    adjusted_thruster_dist2CG = thruster_dist2CG / 1000;

    % Define thruster contribution vectors
    Vec1 = [-1; -1;  0;  0;  1;  1;  0;  0]; % X-component
    Vec2 = [ 0;  0;  1;  1;  0;  0; -1; -1]; % Y-component
    Vec3 = adjusted_thruster_dist2CG;        % Moment arm (Z)

    % Combine vectors into the H matrix structure
    Mat1 = [Vec1, Vec2, Vec3]';
    
    % Adjust thruster forces with decay factor
    F_thrusters = [F_X_nominal; F_X_nominal; F_Y_nominal; F_Y_nominal; 
                   F_X_nominal; F_X_nominal; F_Y_nominal; F_Y_nominal] * thrust_decay_factor;

    % Scale forces for H matrix
    Mat2 = diag(F_thrusters);

    % Compute final H matrix
    H = Mat1 * Mat2;
end

function [thrust_decay_factor, count] = check_thrust_decay(PWMs)
    % Updates the thrust decay factor based on current duty cycles
    %
    % Inputs:
    %   PWMs - Current duty cycle values (vector)
    %
    % Outputs:
    %   thrust_decay_factor - Updated decay factor (scalar)
    %   count - Number of active thrusters (scalar)

    % Normalize PWMs if necessary
    if max(PWMs) > 1
        PWMs = PWMs / max(PWMs);
    end

    % Count active thrusters
    count = sum(PWMs > 0);
    
    % Compute average duty cycle for active thrusters
    average_duty_cycle_per_thruster = sum(max(PWMs, 0)) / max(count, 1);

    % Update thrust decay factor based on average duty cycle
    if average_duty_cycle_per_thruster < 0.3 || count == 0
        thrust_decay_factor = 1;
    else
        thrust_decay_factor = max(0.6 - 2 * average_duty_cycle_per_thruster + 1, 0.5);
    end
end

== matlab function SMPC_safeconstr/Stochastic Model Predictive Control/Unscented Kalman Filter (OBSTACLE)/Unscented Kalman Filter ==
  data: x_0 input; P_0 input; z input; x_est output; P_est output; baseRate parameter; Q_k parameter; R_k parameter; lambda parameter; w_m parameter; w_c parameter
function [x_est, P_est] = fcn(x_0, P_0, z, baseRate, Q_k, R_k, lambda, w_m, w_c)
    % Define dynamics model (using forward euler integration)
    dynamics = @(x, dt) x + dt.*[x(4:6); zeros(3,1)];

    % Define measurement model
    measure = @(x) x(1:3);

    % Run a step of the UKF
    [x_est, P_est] = estimate_UKF(x_0, P_0, z, baseRate, dynamics, measure, ...
                                  6, Q_k, R_k, lambda, w_m, w_c, 3);
end

%% Unscented Kalman Filter Estimation
function [x_est, P_est] = estimate_UKF(x_0, P_0, z, dt, dynamics_fcn, measure_fcn, N, Q, R, lambda, w_m, w_c, d_max)
    % Compute the cholesky decomposition
    L = chol((N + lambda)*P_0)';
    
    % Place sigma points
    X = [x_0, x_0 + L, x_0 - L];
    
    % Propogate sigma points through the dynamics model
    X_plus = zeros(size(X));
    for i = 1:size(X,2)
        X_plus(:,i) = dynamics_fcn(X(:,i), dt);
    end

    % Compute the predicted state and covariance
    x_bar = X_plus*w_m';
    P_bar = (X_plus - x_bar)*diag(w_c)*(X_plus - x_bar)' + Q;

    % Transfer sigma points into the measurement space
    Z = zeros(size(z,1), size(X,2));
    for i = 1:size(X,2)
        Z(:,i) = measure_fcn(X_plus(:,i));
    end

    % Compute the predicted measurement
    z_bar = Z*w_m';

    % Compute measurement covariance and state-measurement cross-covariance
    P_zz = (Z - z_bar)*diag(w_c)*(Z - z_bar)' + R;
    P_xz = (X_plus - x_bar)*diag(w_c)*(Z - z_bar)';

    % Compute the residue
    y = z - z_bar;

    if anynan(z) || all(z == 0) || y'*P_zz*y >= d_max^2
        % If there is no measurement, or it is an outlier, use prediction only
        x_est = x_bar;
        P_est = P_bar;
    else
        % Compute the kalman gain
        K = P_xz/P_zz;

        % Compute estimated state and covariance
        x_est = x_bar + K*y;
        P_est = P_bar - K*P_zz*K';
    end
end

== matlab function SMPC_safeconstr/Thruster Control Code/Change BLUE Behavior/Calculate Duty Cycle/Rotate Forces to Inertial/Create Rotation Matrix ==
  data: Rz input; C_Ib output
function C_Ib = RotateFrame(Rz)

C_bI = [  cos(Rz) sin(Rz)
         -sin(Rz) cos(Rz) ];

C_Ib = inv(C_bI);

end

== matlab function SMPC_safeconstr/Thruster Control Code/Change BLUE Behavior/Rotate Forces to Body/Create Rotation Matrix ==
  data: Rz input; C_bI output
function C_bI = RotateFrame(Rz)

C_bI = [  cos(Rz) sin(Rz)
         -sin(Rz) cos(Rz) ];

end

== matlab function SMPC_safeconstr/Thruster Control Code/Change RED Behavior/Calculate Duty Cycle/Generate Initial Guess/MATLAB Function ==
  data: H output; thruster_dist2CG_RED parameter; F_thrusters_RED parameter
function H = MakeH(thruster_dist2CG_RED,F_thrusters_RED)

    Vec1 = [ -1
             -1
              0 
              0
              1
              1
              0
              0 ];
          
    Vec2 = [  0
              0
              1
              1
              0
              0
             -1
             -1 ];
         
    Vec3 = thruster_dist2CG_RED./1000;
    
    Mat1 = [Vec1, Vec2, Vec3]';
    
    Mat2 = diag((F_thrusters_RED./2));
    
    H    = Mat1*Mat2;

end
